simulink model "TestChaineAirNew"  (R2024b)
settings: Solver=ode45  StartTime=0.0  StopTime=SimuPumpStop  FixedStep=0.1  MaxStep=0.005  RelTol=1e-9  EnableMultiTasking=on
undefined symbols (not defined in the file): AirMotTest, AirPapTest, AirPressureTest, AirTimeTest, gam, nv_remp, Pamb, PcolPapTest, PRcrit, Rair, RegimeTest, SectionPapTest, Tamb, TempsPapTest, TempsTest, Vcol, Vcyl
settings Model: Creator=a030141  LastModifiedBy=ramse
settings SolverCC: AlgebraicLoopSolver=TrustRegion
settings DataIOCC: LimitDataPoints=on  SaveFormat=Array  SignalLoggingSaveFormat=ModelDataLogs  ReturnWorkspaceOutputs=off  SignalLoggingName=sigsOut
settings OptimizationCC: InitFltsAndDblsToZero=on  LifeSpan=inf
settings DebuggingCC: SaveWithParameterizedLinksMsg=none  UnderspecifiedInitializationDetection=Classic  MergeDetectMultiDrivingBlocksExec=none  SignalResolutionControl=TryResolveAllWithWarning  MultiTaskDSMMsg=warning  MultiTaskCondExecSysMsg=none  FcnCallInpInsideContextMsg=warning  UnconnectedInputMsg=warning  UnconnectedOutputMsg=warning  UnconnectedLineMsg=warning  SFUnexpectedBacktrackingDiag=warning  SFNoUnconditionalDefaultTransitionDiag=warning  SFExecutionAtInitializationDiag=none  ArithmeticOperatorsInVariantConditions=warning
settings HardwareCC: ProdBitPerPointer=32  ProdBitPerSizeT=32  ProdBitPerPtrDiffT=32  ProdLargestAtomicFloat=None  ProdIntDivRoundTo=Undefined  ProdEndianess=Unspecified  ProdWordSize=32  ProdHWDeviceType=32-bit Generic  TargetUnknown=on
settings ModelReferenceCC: PropagateSignalLabelsOutOfModel=off
settings RTWCC: GPUComputeCapability=3.5
settings CodeAppCC: StateflowObjectComments=on
settings GRTTargetCC: TargetFcnLib=ansi_tfl_tmw.mat  TargetLangStandard=C89/C90 (ANSI)  CombineOutputUpdateFcns=off  GRTInterface=on
settings ConfigComp: CovMetricSettings=dw  CovSaveCumulativeToWorkspaceVar=on  CovSaveSingleToWorkspaceVar=on

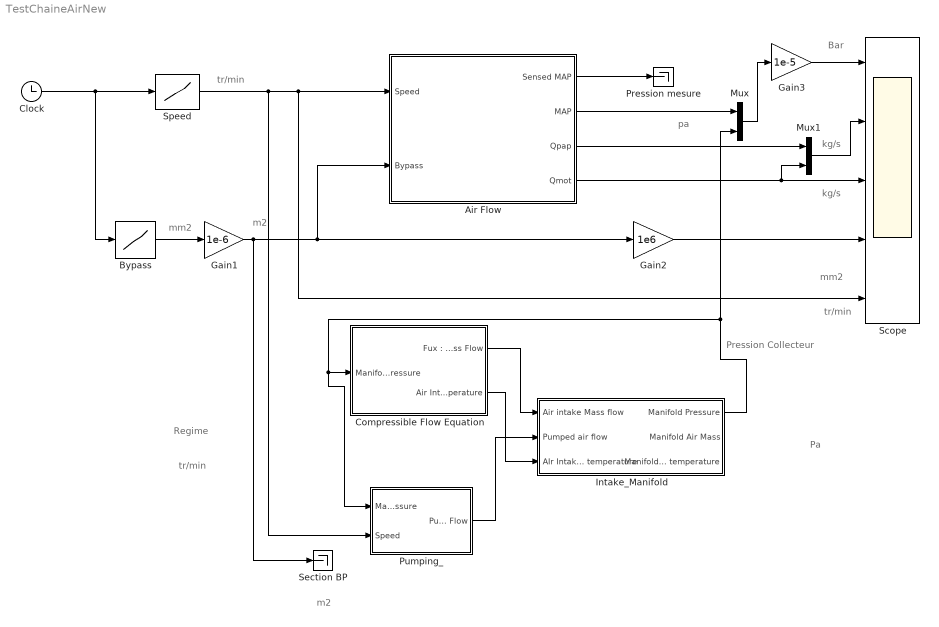
== system TestChaineAirNew ==
  note: Regime
  note: Pression Collecteur
  note: pa
  note: Bar
  note: tr/min
  note: tr/min
  note: m2
  note: tr/min
  note: Pa
  note: m2
  note: mm2
  note: mm2
  note: kg/s
  note: kg/s
  Air Flow : Subsystem
  Bypass : Lookup  InputValues=TempsPapTest  Table=SectionPapTest.*PcolPapTest
  Clock : Clock
  Compressible Flow Equation : Subsystem
  Gain1 : Gain  Gain=1e-6  SaturateOnIntegerOverflow=on  OutDataTypeStr=Inherit: Same as input  ParamDataTypeStr=Inherit: Same as input
  Gain2 : Gain  Gain=1e6  SaturateOnIntegerOverflow=on  OutDataTypeStr=Inherit: Same as input  ParamDataTypeStr=Inherit: Same as input
  Gain3 : Gain  Gain=1e-5  SaturateOnIntegerOverflow=on  OutDataTypeStr=Inherit: Same as input  ParamDataTypeStr=Inherit: Same as input
  Intake_Manifold : Subsystem
  Mux : Mux  Inputs=2
  Mux1 : Mux  Inputs=2
  Pression mesure : Terminator
  Pumping_ : Subsystem
  Scope : Scope  NumInputPorts=5
  Section BP : Terminator
  Speed : Lookup  InputValues=TempsTest  Table=RegimeTest
  wires:
  Speed/1 -> Pumping_/2(Speed), Scope/5, Air Flow/1(Speed)
  Intake_Manifold/1(Manifold Pressure) -> Pumping_/1(Manifold Pressure), Compressible Flow Equation/1(Manifold Pressure), Mux/2
  Clock/1 -> Speed/1, Bypass/1
  Bypass/1 -> Gain1/1
  Gain1/1 -> Section BP/1, Gain2/1, Air Flow/2(Bypass)
  Air Flow/2(MAP) -> Mux/1
  Mux/1 -> Gain3/1
  Gain3/1 -> Scope/1
  Air Flow/4(Qmot) -> Scope/3, Mux1/2
  Gain2/1 -> Scope/4
  Air Flow/3(Qpap) -> Mux1/1
  Mux1/1 -> Scope/2
  Air Flow/1(Sensed MAP) -> Pression mesure/1
  Pumping_/1(Pumped Air Flow) -> Intake_Manifold/2(Pumped air flow)
  Compressible Flow Equation/2(Air Intake Temperature) -> Intake_Manifold/3(AIr Intake temperature)
  Compressible Flow Equation/1("Fux : Air Intake Mass Flow") -> Intake_Manifold/1(Air intake Mass flow)

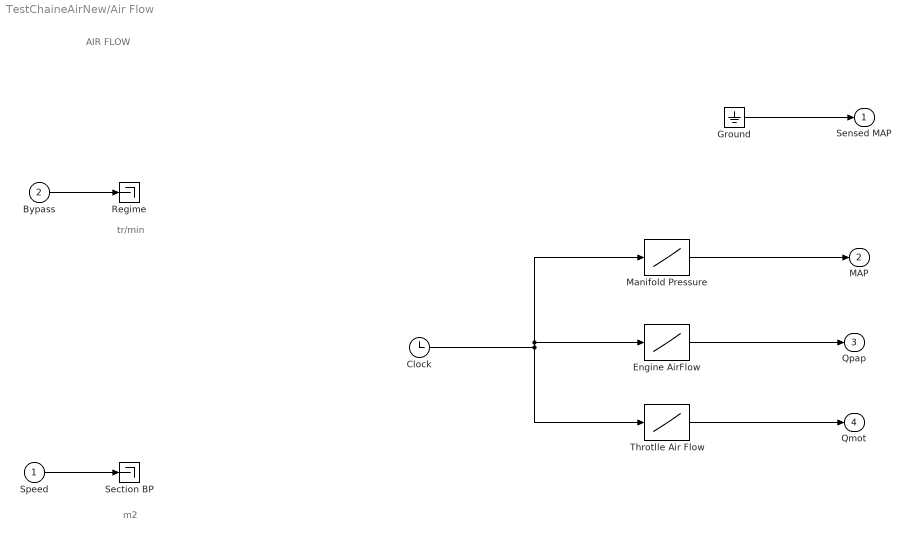
== system TestChaineAirNew/Air Flow ==
  note: AIR FLOW
  note: m2
  note: tr/min
  Speed : Inport
  Bypass : Inport  Port=2
  Clock : Clock
  Engine AirFlow : Lookup  InputValues=AirTimeTest  Table=AirMotTest
  Ground : Ground
  Manifold Pressure : Lookup  InputValues=AirTimeTest  Table=AirPressureTest
  Regime : Terminator
  Section BP : Terminator
  Throtlle Air Flow : Lookup  InputValues=AirTimeTest  Table=AirPapTest
  Sensed MAP : Outport
  MAP : Outport  Port=2
  Qpap : Outport  Port=3
  Qmot : Outport  Port=4
  wires:
  Bypass/1 -> Regime/1
  Speed/1 -> Section BP/1
  Ground/1 -> Sensed MAP/1
  Clock/1 -> Manifold Pressure/1, Engine AirFlow/1, Throtlle Air Flow/1
  Manifold Pressure/1 -> MAP/1
  Throtlle Air Flow/1 -> Qmot/1
  Engine AirFlow/1 -> Qpap/1

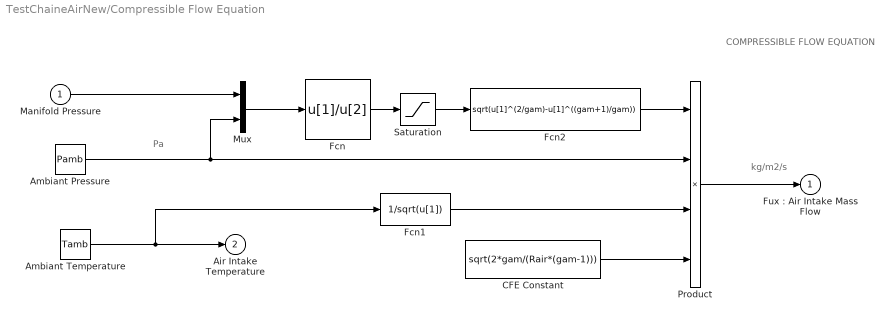
== system TestChaineAirNew/Compressible Flow Equation ==
  note: COMPRESSIBLE FLOW EQUATION
  note: Pa
  note: kg/m2/s
  Manifold Pressure : Inport
  Ambiant Pressure : Constant  Value=Pamb
  Ambiant Temperature : Constant  Value=Tamb
  "CFE Constant " : Constant  Value=sqrt(2*gam/(Rair*(gam-1)))
  Fcn : Fcn  Expr=u[1]/u[2]
  Fcn1 : Fcn  Expr=1/sqrt(u[1])
  Fcn2 : Fcn  Expr=sqrt(u[1]^(2/gam)-u[1]^((gam+1)/gam))
  Mux : Mux  Inputs=2
  Product : Product  Inputs=4  InputSameDT=on  SaturateOnIntegerOverflow=on  OutDataTypeStr=Inherit: Same as first input
  Saturation : Saturate  UpperLimit=1  LowerLimit=PRcrit
  "Fux : Air Intake Mass Flow" : Outport
  Air Intake Temperature : Outport  Port=2
  wires:
  Ambiant Pressure/1 -> Product/2, Mux/2
  Product/1 -> "Fux : Air Intake Mass Flow"/1
  "CFE Constant "/1 -> Product/4
  Fcn2/1 -> Product/1
  Saturation/1 -> Fcn2/1
  Fcn1/1 -> Product/3
  Fcn/1 -> Saturation/1
  Mux/1 -> Fcn/1
  Manifold Pressure/1 -> Mux/1
  Ambiant Temperature/1 -> Fcn1/1, Air Intake Temperature/1

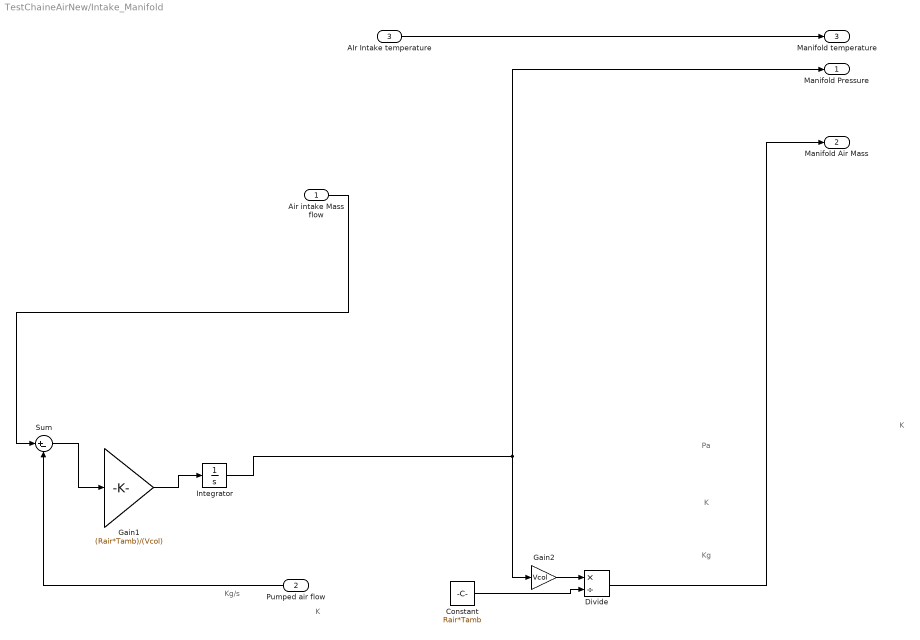
== system TestChaineAirNew/Intake_Manifold ==
  note: Kg/s
  note: Kg
  note: K
  note: Pa
  note: K
  note: K
  Air intake Mass flow : Inport
  Pumped air flow : Inport  Port=2
  AIr Intake temperature : Inport  Port=3
  Constant : Constant  Value=Rair*Tamb
  Divide : Product  Inputs=*/
  Gain1 : Gain  Gain=(Rair*Tamb)/(Vcol)
  Gain2 : Gain  Gain=Vcol
  Integrator : Integrator
  Sum : Sum  Inputs=|+-
  Manifold Pressure : Outport
  Manifold Air Mass : Outport  Port=2
  Manifold temperature : Outport  Port=3
  wires:
  Gain2/1 -> Divide/1
  Air intake Mass flow/1 -> Sum/1
  Sum/1 -> Gain1/1
  Divide/1 -> Manifold Air Mass/1
  Gain1/1 -> Integrator/1
  Pumped air flow/1 -> Sum/2
  Constant/1 -> Divide/2
  Integrator/1 -> Manifold Pressure/1, Gain2/1
  AIr Intake temperature/1 -> Manifold temperature/1

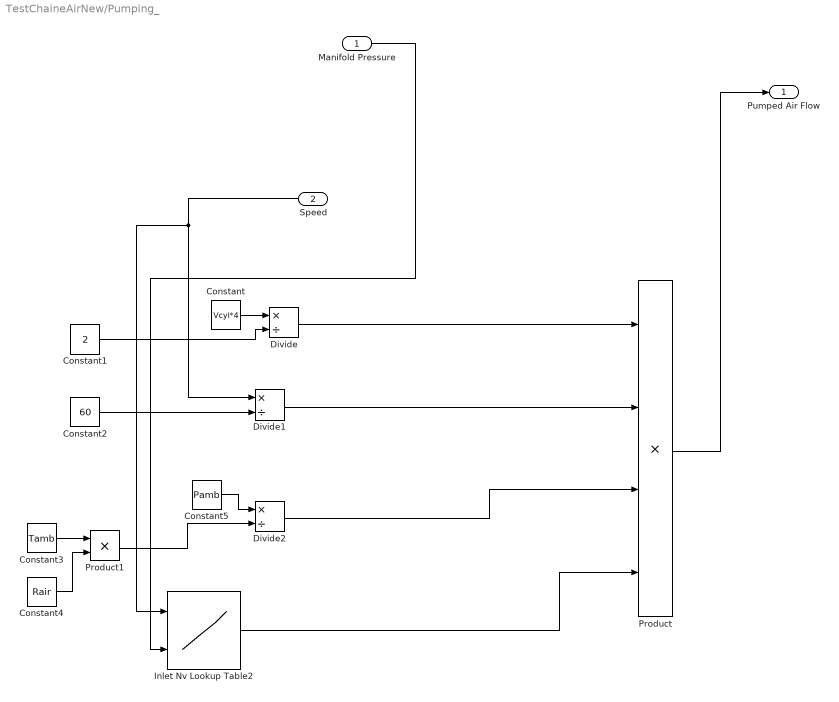
== system TestChaineAirNew/Pumping_ ==
  Manifold Pressure : Inport
  Speed : Inport  Port=2
  Constant : Constant  Value=Vcyl*4
  Constant1 : Constant  Value=2
  Constant2 : Constant  Value=60
  Constant3 : Constant  Value=Tamb
  Constant4 : Constant  Value=Rair
  Constant5 : Constant  Value=Pamb
  Divide : Product  Inputs=*/
  Divide1 : Product  Inputs=*/
  Divide2 : Product  Inputs=*/
  Inlet Nv Lookup Table2 : Lookup2D  RowIndex=Ne_remp  ColumnIndex=Pcol_remp  Table=nv_remp
  Product : Product  Inputs=4
  Product1 : Product
  Pumped Air Flow : Outport
  wires:
  Constant3/1 -> Product1/1
  Constant5/1 -> Divide2/1
  Divide/1 -> Product/1
  Constant/1 -> Divide/1
  Divide2/1 -> Product/3
  Divide1/1 -> Product/2
  Product1/1 -> Divide2/2
  Inlet Nv Lookup Table2/1 -> Product/4
  Constant1/1 -> Divide/2
  Constant2/1 -> Divide1/2
  Constant4/1 -> Product1/2
  Product/1 -> Pumped Air Flow/1
  Speed/1 -> Inlet Nv Lookup Table2/1, Divide1/1
  Manifold Pressure/1 -> Inlet Nv Lookup Table2/2
